simulink library "sensorToolsLib"  (R2023b)
settings: Solver=VariableStepAuto  StartTime=0.0  StopTime=10.0  RelTol=1e-3
settings Model: Creator=kristopherriordan  LastModifiedBy=kristopherriordan

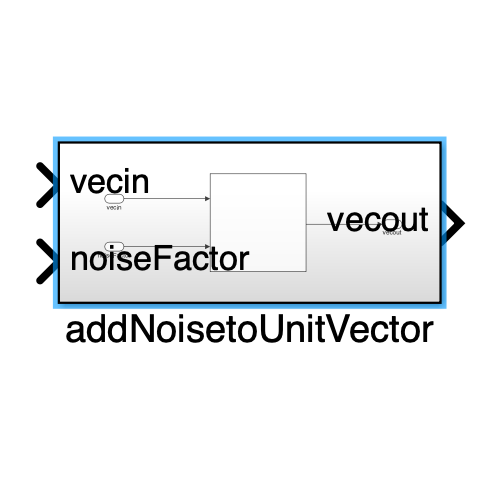
[thumbnail: Simulink's stored preview of the top-level diagram]
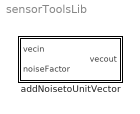
== system sensorToolsLib ==
  addNoisetoUnitVector : Subsystem

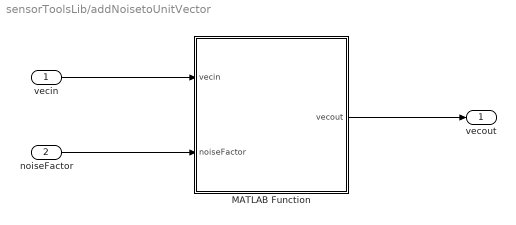
== system sensorToolsLib/addNoisetoUnitVector ==
  vecin : Inport
  noiseFactor : Inport  Port=2
  MATLAB Function : MATLAB Function  TreatAsAtomicUnit=on
  vecout : Outport
  wires:
  vecin/1 -> MATLAB Function/1(vecin)
  noiseFactor/1 -> MATLAB Function/2(noiseFactor)
  MATLAB Function/1(vecout) -> vecout/1

== matlab function sensorToolsLib/addNoisetoUnitVector/MATLAB Function ==
  data: vecin input; vecout output size=size(vecin); noiseFactor input size=1
function vecout = perturbUnitVectors(vecin, noiseFactor)

vecout = zeros(size(vecin));

dim = size(vecin);

pert = noiseFactor.*(2.*rand(dim) - 1);

vecout = vecin + pert;

for i=1:dim(2)
    vecout(:,i) = vecout(:,i)./norm(vecout(:,i));
end
